simulink model "DragModelMomentDragNew"  (R2017b)
settings: Solver=VariableStepAuto  StartTime=0.0  StopTime=10.0  RelTol=1e-3  EnableMultiTasking=on
undefined symbols (not defined in the file): Aero, Uav
settings Model: Creator=jban039  LastModifiedBy=jban039
settings DataIOCC: LimitDataPoints=on
settings OptimizationCC: LifeSpan=inf
settings DebuggingCC: AllowSymbolicDim=off  SFUnexpectedBacktrackingDiag=warning  SFNoUnconditionalDefaultTransitionDiag=warning  SFExecutionAtInitializationDiag=none
settings ModelReferenceCC: PropagateSignalLabelsOutOfModel=off
settings CodeAppCC: StateflowObjectComments=on
settings GRTTargetCC: TargetLangStandard=C89/C90 (ANSI)
settings ConfigComp: CovMetricSettings=dw  CovHtmlReporting=on  CovSaveCumulativeToWorkspaceVar=on  CovSaveSingleToWorkspaceVar=on  CovExternalEMLEnable=off

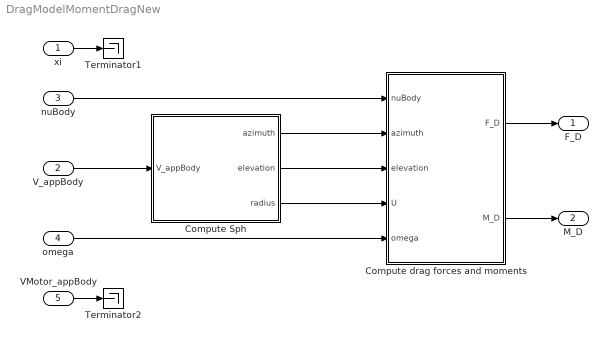
== system DragModelMomentDragNew ==
  xi : Inport  Unit=m  PortDimensions=3
  V_appBody : Inport  Port=2  Unit=m/s  PortDimensions=3
  nuBody : Inport  Port=3  Unit=rad/s  PortDimensions=3
  omega : Inport  Port=4  Unit=rad/s  PortDimensions=Uav.N_ROTORS
  VMotor_appBody : Inport  Port=5  Unit=m/s  PortDimensions=[3,4]
  Compute Sph : MATLAB Function  TreatAsAtomicUnit=on
  Compute drag forces and moments : MATLAB Function  TreatAsAtomicUnit=on
  Terminator1 : Terminator
  Terminator2 : Terminator
  F_D : Outport  Unit=N
  M_D : Outport  Port=2  Unit=N*m
  wires:
  Compute drag forces and moments/1(F_D) -> F_D/1
  xi/1 -> Terminator1/1
  omega/1 -> Compute drag forces and moments/5(omega)
  nuBody/1 -> Compute drag forces and moments/1(nuBody)
  Compute Sph/3(radius) -> Compute drag forces and moments/4(U)
  Compute Sph/2(elevation) -> Compute drag forces and moments/3(elevation)
  Compute Sph/1(azimuth) -> Compute drag forces and moments/2(azimuth)
  VMotor_appBody/1 -> Terminator2/1
  Compute drag forces and moments/2(M_D) -> M_D/1
  V_appBody/1 -> Compute Sph/1(V_appBody)

== matlab function DragModelMomentDragNew/Compute Sph ==
  data: V_appBody input; azimuth output; elevation output; radius output
function [azimuth, elevation, radius] = computeSph(V_appBody)
%#codegen

% Convert from polar to spherical coordinates
[ azimuth, elevation, radius ] = cart2sph( V_appBody(1), V_appBody(2), V_appBody(3) );

== matlab function DragModelMomentDragNew/Compute drag forces and moments ==
  data: nuBody input; azimuth input; elevation input; U input; omega input; F_D output; M_D output; Uav parameter; Aero parameter
function [F_D, M_D] = computeDrag( nuBody, azimuth, elevation, U, ...
                                   omega, Uav, Aero )
%#codegen
alpha = -elevation;

% Outputs
F_D = zeros(3,1);
M_D = zeros(3,1);

if strcmp( Aero.Type, 'Body oriented' )
    Cz1 = dot( Aero.Cz1.coefs, [1, alpha] ); % modify
    Cx1 = dot( Aero.Cx1.coefs, [1, cos(8*alpha)] ); % modify
    Fz_lift = 0.5 .* Uav.RHO_AIR .* U^2 .* Cz1 * Uav.A_UAV;
    Fx_drag = 0.5 .* Uav.RHO_AIR .* U^2 .* Cx1 * Uav.A_UAV;
    F_D = [Fx_drag*cos(alpha); Fx_drag*sin(alpha); Fz_lift];
else
    x1 = cos(-elevation);
    x2 = mean(omega);
    Cd1 = dot( Aero.Cd1.coefs, [ 1, x1, x2, x1*x2, x1^2, x2^2, x1^2*x2^2  ] );
    Cd2 = dot( Aero.Cd2.coefs, [ 1, x1, x2, x1*x2, x1^2, x2^2, x1^2*x2^2  ] );

    f_D = 0.5 * Uav.RHO_AIR * Cd1 * U^2 + ...
        0.5 * Uav.RHO_AIR * Cd2 * U;
    F_D = zeros(3,1);

    x1 = -elevation;
    x2 = 0;
    Cl = dot( Aero.Cl.coefs, [ 1, x1, x2, x1*x2, x1^2, x2^2, x1^2*x2^2  ] );

    f_l = 0.5 * Uav.RHO_AIR * Cl * U^2;
    F_l = zeros(3,1);

    [ F_D(1), F_D(2), F_D(3) ] = sph2cart( azimuth, elevation, f_D );
    [ F_l(1), F_l(2), F_l(3) ] = sph2cart( azimuth, elevation + pi/2, f_l );

    F_D = F_D + F_l;

    x1 = sin(-elevation);
    x2 = U;
    CdRot1 = dot( Aero.CdRot1.coefs, [ 1, x1, x2, x1*x2, x1^2, x2^2, x1^2*x2^2  ] );
    CdRot2 = dot( Aero.CdRot2.coefs, [ 1, x1, x2, x1*x2, x1^2, x2^2, x1^2*x2^2  ] );

    m_D = CdRot1 * mean(omega)^2 + CdRot2 * mean(omega);

    M_D = zeros(3,1);
    [ M_D(1), M_D(2), M_D(3) ] = sph2cart( azimuth+pi/2, 0, m_D );
end

% Drag moment, applied to independent axes
% M_D = M_D + 0.5 * Uav.RHO_AIR * Uav.C_DM * ( norm(nuBody) .* nuBody );
% M_D = M_D;
